simulink model "delay"  (R2015b)
settings: Solver=ode45  StartTime=0.0  StopTime=10.0  RelTol=1e-3
settings Model: Creator=Django  LastModifiedBy=exbot
settings DataIOCC: SaveFormat=Array
settings DebuggingCC: SolverPrmCheckMsg=warning
settings HardwareCC: ProdBitPerPointer=32  ProdLargestAtomicFloat=None  ProdIntDivRoundTo=Undefined  ProdEndianess=Unspecified  ProdWordSize=32  ProdHWDeviceType=32-bit Generic
settings GRTTargetCC: GeneratePreprocessorConditionals=Disable all
settings ConfigComp: CovModelRefEnable=Off  CovSFcnEnable=off

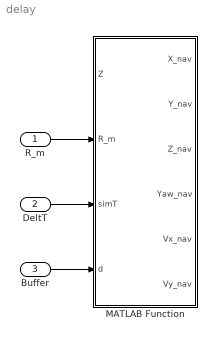
== system delay ==
  R_m : Inport
  DeltT : Inport  Port=2
  Buffer : Inport  Port=3
  MATLAB Function : MATLAB Function  TreatAsAtomicUnit=on
  wires:
  R_m/1 -> MATLAB Function/2(R_m)
  DeltT/1 -> MATLAB Function/3(simT)
  Buffer/1 -> MATLAB Function/4(d)
  ? -> MATLAB Function/1(Z)

== matlab function delay/MATLAB Function ==
  data: X_nav output; Z input; Y_nav output; Z_nav output; Yaw_nav output; Vx_nav output; Vy_nav output; R_m input; simT input; d input
function [X_nav,Y_nav,Z_nav,Yaw_nav,Vx_nav,Vy_nav] = fcn(Z,R_m,simT,d)
persistent Phi;
if isempty(Phi)
    Phi = [0 0 0 1 0 0 0;
           0 0 0 0 1 0 0;
           0 0 0 0 0 1 0;
           0 0 0 0 0 0 0;
           0 0 0 0 0 0 0;
           0 0 0 0 0 0 0;
           0 0 0 0 0 0 0];
end

persistent Tao;
if isempty(Tao)
    Tao = [0 0 0 0 0 0 0;
           0 0 0 0 0 0 0;
           0 0 0 0 0 0 0;
           0 0 0 1 0 0 0;
           0 0 0 0 1 0 0;
           0 0 0 0 0 1 0;
           0 0 0 0 0 0 1];
end

persistent Q;
if isempty(Q)
    Q = 500;
end

persistent H;
if isempty(H)
    H = [1 0 0 0 0 0 0;
         0 1 0 0 0 0 0;
         0 0 1 0 0 0 0;
         0 0 0 1 0 0 0;
         0 0 0 0 1 0 0;
         0 0 0 0 0 0 1];
end

persistent R;
if isempty(R)
    R = zeros(6,6);
    for i = 1:6
        R(i,i) = R_m(i);
    end
end

persistent Xe;
if isempty(Xe)
    Xe = [0 0 0 0 0 0 0]';
end

persistent X_e;
if isempty(X_e)
    X_e = zeros(7,5);
end

persistent Z_e;
if isempty(Z_e)
    Z_e = zeros(6,5);
end

persistent P;
if isempty(P)
    P = Q*diag([1 1 1 1 1 1 1]); % 估计误差协方差阵
end

persistent P_;
if isempty(P_)
    P_ = zeros(7,7,5); % 估计误差协方差阵
    for i=1:d
        P_(:,:,i) = P;
    end
end

% 状态变量的先验估计
X_e(:,d) = (eye(7)+simT*Phi)*Xe;
% 观测向量的先验估计
Z_e(:,d) = H*X_e(:,d);
% 计算先验估计误差协方差阵
P_(:,:,d) = Phi*P*Phi'+Tao*Q*Tao';

% 观测值 [x y z vx vy yaw]'  输入Z=[x y z pitch yaw roll vx vy vz]'
Zm = [Z(1)/1000 Z(2)/1000 Z(3)/1000 Z(7)/1000 Z(8)/1000 Z(5)]';

% 计算卡尔曼增益
Kk = P_(:,:,1)*H'*(inv(H*P_(:,:,1)*H'+R));
% 计算后验估计
Xe = X_e(:,1)+Kk*(Zm-Z_e(:,1));
% 计算后验协方差阵
P=(eye(7)-Kk*H)*P_(:,:,1);

% 更新缓冲区
X_e(:,1:d-1) = X_e(:,2:d);
Z_e(:,1:d-1) = Z_e(:,2:d);
P_(:,:,1:d-1) = P_(:,:,2:d);

% 往前预测直到当前时刻
for i=1:d
    Xe = Xe+simT*Phi*Xe;  
end
X_nav = Xe(1);
Y_nav = Xe(2);
Z_nav = Xe(3);
Yaw_nav = Xe(7);
Vx_nav = Xe(4);
Vy_nav = Xe(5);
end
